simulink model "HW3_sim_v3b_backup"  (R2022b)
settings: Solver=VariableStepAuto  StartTime=0.0  StopTime=1000  RelTol=1e-3
values from neighbouring files (symbols this model uses):
  A = 4*1e-4    (= 0.0004)    [Variables.m]    (also in vars.m)
  e_op = i_op*R    [vars.m]
  g = 5*1e-4    (= 0.0005)    [Variables.m]    (also in vars.m)
  i_op = sqrt(2*K_s*(x_i-x_op)*(x_op+g)^2/(N^2*mu_0*A))    [vars.m]
  m = 0.05    [Variables.m]    (also in vars.m)
  N = 100    [Variables.m]    (also in vars.m)
  R = 1    [Variables.m]    (also in vars.m)
  v_op = 0    [vars.m]
  x_i = 1e-2    (= 0.01)    [Variables.m]    (also in vars.m)
  x_op = x_ops(x_opNum)    [vars.m]
undefined symbols (not defined in the file or in its folder): f_d, fre, k_s, u_o
settings Model: Creator=Yuxiong  LastModifiedBy=Yuxiong
settings SolverCC: MaxConsecutiveMinStep=2  ShapePreserveControl=EnableAll

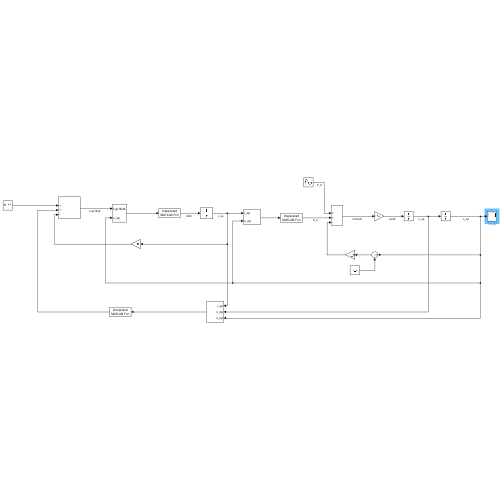
[thumbnail: Simulink's stored preview of the top-level diagram]
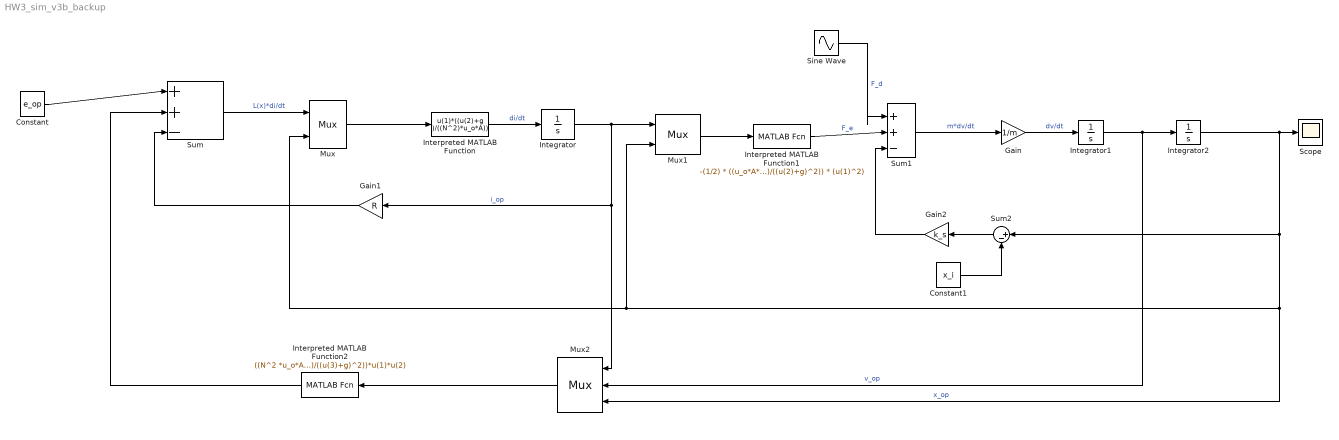
== system HW3_sim_v3b_backup ==
  Constant : Constant  Value=e_op
  Constant1 : Constant  Value=x_i
  Gain : Gain  Gain=1/m
  Gain1 : Gain  Gain=R
  Gain2 : Gain  Gain=k_s
  Integrator : Integrator  InitialCondition=i_op
  Integrator1 : Integrator  InitialCondition=v_op
  Integrator2 : Integrator  InitialCondition=x_op
  Interpreted MATLAB Function : MATLABFcn  MATLABFcn=u(1)*((u(2)+g )/((N^2)*u_o*A))
  Interpreted MATLAB Function1 : MATLABFcn  MATLABFcn=-(1/2) * ((u_o*A*N^2)/((u(2)+g)^2)) * (u(1)^2)
  Interpreted MATLAB Function2 : MATLABFcn  MATLABFcn=((N^2 *u_o*A)/((u(3)+g)^2))*u(1)*u(2)
  Mux : Mux  Inputs=2
      settings: DisplayOption=signals
  Mux1 : Mux  Inputs=2
      settings: DisplayOption=signals
  Mux2 : Mux  Inputs=3
      settings: DisplayOption=signals
  Scope : Scope
  Sine Wave : Sin  Amplitude=f_d  Frequency=2*pi*fre  SampleTime=0
  Sum : Sum  Inputs=|++-
  Sum1 : Sum  Inputs=|++-
  Sum2 : Sum  Inputs=|+-
  wires:
  Constant/1 -> Sum/1
  Sum/1 -> Mux/1  "L(x)*di/dt"
  Mux/1 -> Interpreted MATLAB Function/1
  Interpreted MATLAB Function/1 -> Integrator/1  "di/dt"
  Integrator/1 -> Gain1/1, Mux2/1, Mux1/1  "i_op"
  Mux1/1 -> Interpreted MATLAB Function1/1
  Interpreted MATLAB Function1/1 -> Sum1/2  "F_e"
  Sum1/1 -> Gain/1  "m*dv/dt"
  Gain/1 -> Integrator1/1  "dv/dt"
  Integrator1/1 -> Mux2/2, Integrator2/1  "v_op"
  Mux2/1 -> Interpreted MATLAB Function2/1
  Integrator2/1 -> Sum2/1, Mux2/3, Mux/2, Mux1/2, Scope/1  "x_op"
  Sine Wave/1 -> Sum1/1  "F_d"
  Interpreted MATLAB Function2/1 -> Sum/2
  Gain1/1 -> Sum/3
  Constant1/1 -> Sum2/2
  Sum2/1 -> Gain2/1
  Gain2/1 -> Sum1/3
